simulink model "Processor"  (R2025b)
settings: Solver=VariableStepAuto  StartTime=0.0  StopTime=inf  RelTol=1e-3
libraries: dspsigops x7, hdlsllib x1
settings Model: Creator=cyber  LastModifiedBy=cyber

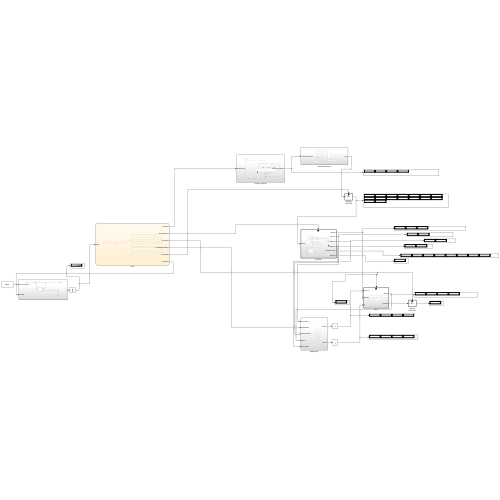
[thumbnail: Simulink's stored preview of the top-level diagram]
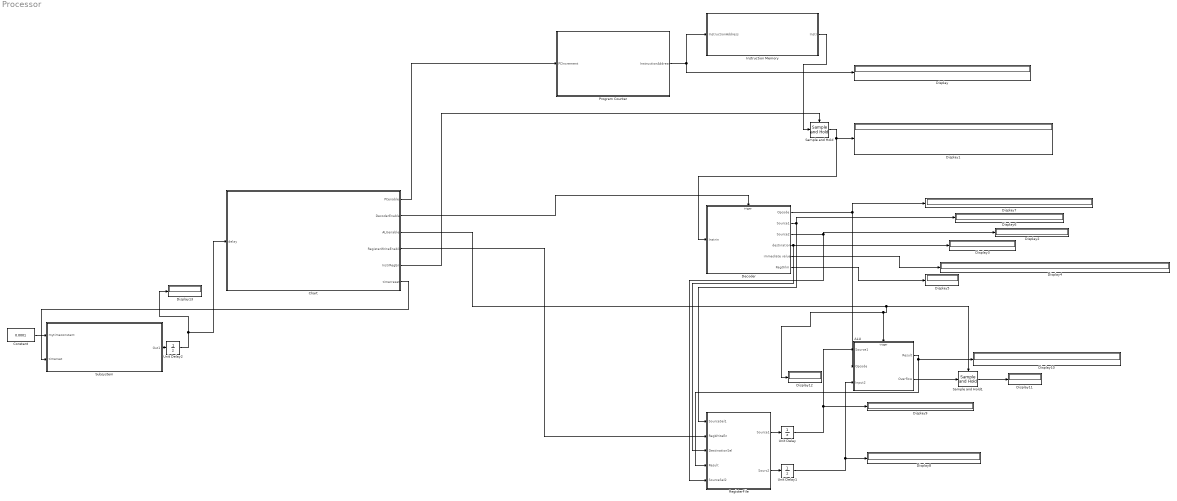
== system Processor ==
  ALU : Subsystem
  Chart : Stateflow chart  TreatAsAtomicUnit=on
  Constant : Constant  Value=0.0001
  Decoder : Subsystem
  Display{,1..13} (14 alike) : Display
  Instruction Memory : Subsystem
  Program Counter : Subsystem
  RegisterFile : Subsystem
  Sample and Hold : dspsigops/Sample and Hold  trig=Rising edge  initCond=0  latchinput=off
  Sample and Hold1 : dspsigops/Sample and Hold  trig=Rising edge  initCond=0  latchinput=off
  Subsystem : Subsystem
  Unit Delay : UnitDelay  SampleTime=-1  HasFrameUpgradeWarning=on
  Unit Delay1 : UnitDelay  SampleTime=-1  HasFrameUpgradeWarning=on
  Unit Delay2 : UnitDelay  SampleTime=-1  HasFrameUpgradeWarning=on
  wires:
  Program Counter/1(InstructionAddress) -> Display/1, Instruction Memory/1(InstructionAddress)
  Instruction Memory/1(Instr) -> Sample and Hold/1
  Sample and Hold/1 -> Decoder/1(Instrin), Display1/1
  Decoder/5(immediate value) -> Display4/1
  Decoder/6(RegOrlm) -> Display5/1
  Decoder/4(destination) -> Display3/1, RegisterFile/3(DestinationSel)
  Decoder/3(Source2) -> RegisterFile/5(SourceSel2), Display2/1
  Decoder/2(Source1) -> RegisterFile/1(SourceSel1), Display6/1
  Decoder/1(Opcode) -> ALU/2(Opcode), Display7/1
  RegisterFile/1(Source1) -> Unit Delay/1
  Unit Delay/1 -> ALU/1(Source1), Display9/1
  RegisterFile/2(Sourc2) -> Unit Delay1/1
  Unit Delay1/1 -> ALU/3(Input2), Display8/1
  ALU/1(Result) -> Display10/1, RegisterFile/4(Result)
  Chart/3(ALUenable) -> Display12/1, ALU/Trigger, Sample and Hold1/Trigger
  ALU/2(Overflow) -> Sample and Hold1/1
  Sample and Hold1/1 -> Display11/1
  Chart/1(PCenable) -> Program Counter/1(PCIncrement)
  Chart/2(DecoderEnable) -> Decoder/Trigger
  Chart/5(InstrRegEn) -> Sample and Hold/Trigger
  Chart/4(RegisterWriteEnable) -> RegisterFile/2(RegWriteEn)
  Subsystem/1(Out1) -> Unit Delay2/1
  Unit Delay2/1 -> Chart/1(delay), Display13/1
  Constant/1 -> Subsystem/1(mytimeconstant)
  Chart/6(timerreset) -> Subsystem/2(timerset)

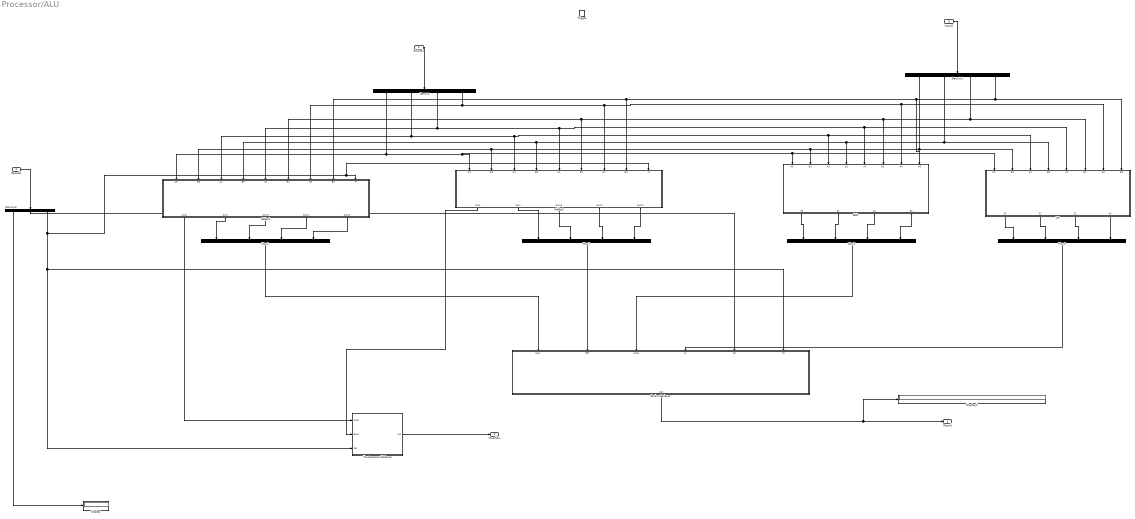
== system Processor/ALU ==
  Source1 : Inport
  Opcode : Inport  Port=2
  Input2 : Inport  Port=3
  Trigger : TriggerPort  VariantControl=(inherit)  PortDimensions=1
  4to1multplexer : Subsystem
  AND : Subsystem
  Adder1 : Subsystem
  Adder2 : Subsystem
  Demux : Demux
  Demux1 : Demux
  Demux2 : Demux  Outputs=3
  Display : Display
  Display1 : Display
  Mux{1..4} (4 alike) : Mux
  OR : Subsystem
  Twotoonemultiplexer : Subsystem
  Result : Outport
  Overflow : Outport  Port=2
  wires:
  Demux2/1 -> Display/1
  Demux1/2 -> OR/4(B2), Adder2/4(B2), Adder1/4(B2), AND/4(B2)
  Mux2/1 -> 4to1multplexer/2(Diff)
  Demux/1 -> Adder1/1(A3), Adder2/1(A3), OR/1(A3), AND/1(A3)
  Adder1/2(Sum) -> Mux1/1
  Demux1/4 -> OR/8(B0), AND/8(B0), Adder2/8(B0), Adder1/8(B0)
  Demux/4 -> Adder1/7(A0), OR/7(A0), AND/7(A0), Adder2/7(A0)
  Demux/2 -> Adder1/3(A2), OR/3(A2), AND/3(A2), Adder2/3(A2)
  Demux1/3 -> OR/6(B1), Adder2/6(B1), Adder1/6(B1), AND/6(B1)
  Demux2/3 -> Adder2/9(M), Adder1/9(M), Twotoonemultiplexer/3(Sel), 4to1multplexer/6(S1)
  Demux1/1 -> OR/2(B3), Adder1/2(B3), Adder2/2(B3), AND/2(B3)
  Demux/3 -> Adder1/5(A1), OR/5(A1), AND/5(A1), Adder2/5(A1)
  Mux4/1 -> 4to1multplexer/4(or)
  Adder2/1(Cout) -> Twotoonemultiplexer/2(Bout)
  Demux2/2 -> 4to1multplexer/5(S0)
  Adder1/3(Sum3) -> Mux1/2
  Mux3/1 -> 4to1multplexer/3(AND)
  Adder1/4(Sum1) -> Mux1/3
  Adder1/1(Cout) -> Twotoonemultiplexer/1(Cout)
  Mux1/1 -> 4to1multplexer/1(Sum)
  Opcode/1 -> Demux2/1
  Twotoonemultiplexer/1(out) -> Overflow/1
  Adder1/5(Sum2) -> Mux1/4
  4to1multplexer/1(out) -> Display1/1, Result/1
  Source1/1 -> Demux/1
  Input2/1 -> Demux1/1
  AND/1(S3) -> Mux3/1
  AND/2(S2) -> Mux3/2
  AND/3(S1) -> Mux3/3
  AND/4(S0) -> Mux3/4
  OR/1(S3) -> Mux4/1
  OR/2(S2) -> Mux4/2
  OR/3(S1) -> Mux4/3
  OR/4(S0) -> Mux4/4
  Adder2/2(Sum) -> Mux2/1
  Adder2/3(Sum3) -> Mux2/2
  Adder2/4(Sum1) -> Mux2/3
  Adder2/5(Sum2) -> Mux2/4

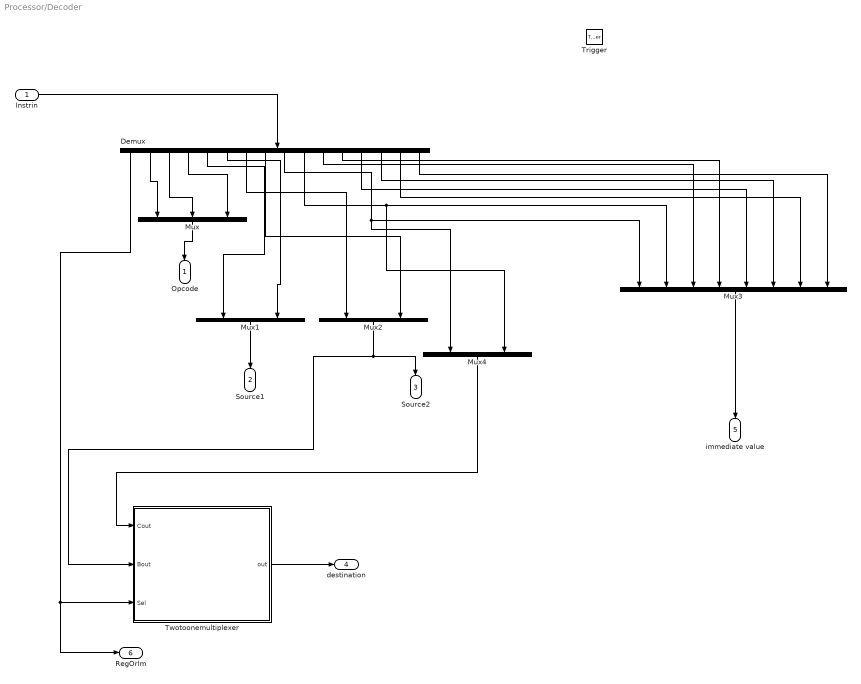
== system Processor/Decoder ==
  Instrin : Inport
  Trigger : TriggerPort  VariantControl=(inherit)  PortDimensions=1
  Demux : Demux  Outputs=16
  Mux : Mux  Inputs=3
  Mux1 : Mux  Inputs=2
  Mux2 : Mux  Inputs=2
  Mux3 : Mux  Inputs=8
  Mux4 : Mux  Inputs=2
  Twotoonemultiplexer : Subsystem
  Opcode : Outport
  Source1 : Outport  Port=2
  Source2 : Outport  Port=3
  destination : Outport  Port=4
  immediate value : Outport  Port=5
  RegOrlm : Outport  Port=6
  wires:
  Demux/12 -> Mux3/4
  Twotoonemultiplexer/1(out) -> destination/1
  Demux/14 -> Mux3/6
  Demux/1 -> RegOrlm/1, Twotoonemultiplexer/3(Sel)
  Mux2/1 -> Source2/1, Twotoonemultiplexer/2(Bout)
  Demux/10 -> Mux4/2, Mux3/2
  Demux/16 -> Mux3/8
  Demux/9 -> Mux4/1, Mux3/1
  Demux/4 -> Mux/3
  Mux4/1 -> Twotoonemultiplexer/1(Cout)
  Demux/8 -> Mux2/2
  Demux/2 -> Mux/1
  Mux3/1 -> immediate value/1
  Demux/7 -> Mux2/1
  Demux/3 -> Mux/2
  Demux/6 -> Mux1/2
  Mux/1 -> Opcode/1
  Mux1/1 -> Source1/1
  Demux/15 -> Mux3/7
  Demux/11 -> Mux3/3
  Demux/13 -> Mux3/5
  Demux/5 -> Mux1/1
  Instrin/1 -> Demux/1

== system Processor/Instruction Memory ==
  InstructionAddress : Inport
  4to1multplexer : Subsystem
  Constant : Constant  Value=[0 0 0 1 0 0 0 1 1 0 0 0 0 0 0 0 ]
  Constant1 : Constant  Value=[0 0 0 0 0 0 0 1 1 0 0 0 0 0 0 0 ]
  Constant2 : Constant  Value=[0 0 0 0 0 0 0 1 1 0 0 0 0 0 0 0 ]
  Constant3 : Constant  Value=[0 0 0 0 0 0 0 1 1 0 0 0 0 0 0 0 ]
  Demux : Demux
  Display : Display
  Display1 : Display
  Display2 : Display
  Instr : Outport
  wires:
  Demux/3 -> 4to1multplexer/5(S0)
  Demux/2 -> Display1/1
  Constant1/1 -> 4to1multplexer/2(2)
  Constant3/1 -> 4to1multplexer/4(4)
  Constant/1 -> 4to1multplexer/1(1)
  4to1multplexer/1(out) -> Instr/1
  Demux/4 -> 4to1multplexer/6(S1)
  Constant2/1 -> 4to1multplexer/3(3)
  InstructionAddress/1 -> Demux/1, Display2/1
  Demux/1 -> Display/1

== system Processor/Program Counter ==
  PCIncrement : Inport
  Adder : Subsystem
  Constant1 : Constant
  Constant2 : Constant  Value=0
  Demux : Demux
  Display : Display
  Mux : Mux
  Program Counter : dspsigops/Sample and Hold  trig=Rising edge  initCond=0  latchinput=off
  Unit Delay : UnitDelay  SampleTime=-1  HasFrameUpgradeWarning=on
  InstructionAddress : Outport
  wires:
  Constant2/1 -> Adder/2(B3), Adder/4(B2), Adder/6(B1), Adder/9(Cin)
  Demux/2 -> Adder/3(A2)
  PCIncrement/1 -> Program Counter/Trigger
  Constant1/1 -> Adder/8(B0)
  Demux/3 -> Adder/5(A1)
  Program Counter/1 -> Demux/1
  Demux/4 -> Adder/7(A0)
  Demux/1 -> Adder/1(A3)
  Adder/2(Sum) -> Mux/1
  Adder/1(Cout) -> Display/1
  Unit Delay/1 -> Program Counter/1
  Mux/1 -> InstructionAddress/1, Unit Delay/1
  Adder/5(Sum2) -> Mux/4
  Adder/3(Sum3) -> Mux/2
  Adder/4(Sum1) -> Mux/3

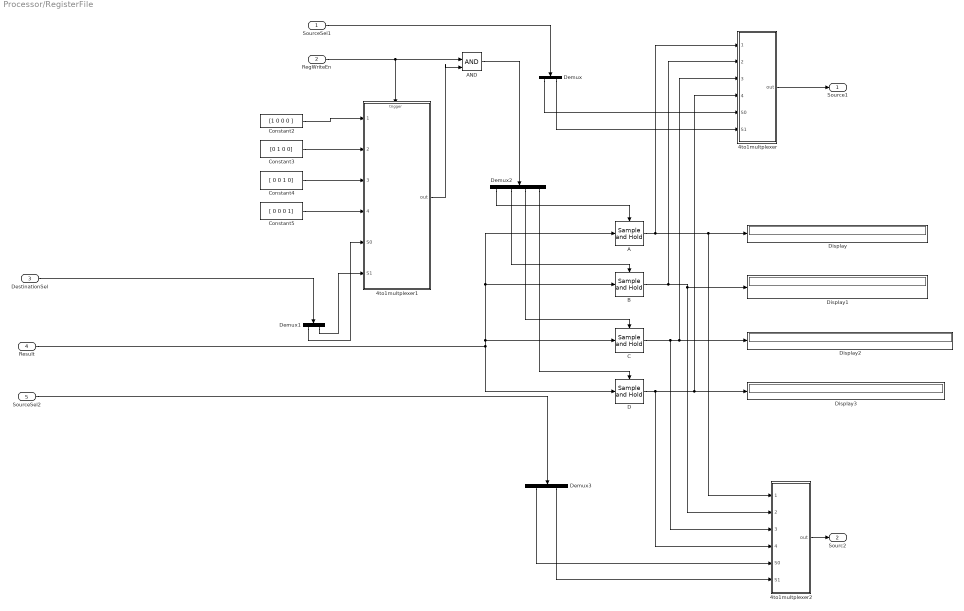
== system Processor/RegisterFile ==
  SourceSel1 : Inport
  RegWriteEn : Inport  Port=2
  DestinationSel : Inport  Port=3
  Result : Inport  Port=4
  SourceSel2 : Inport  Port=5
  4to1multplexer : Subsystem
  4to1multplexer1 : Subsystem
  4to1multplexer2 : Subsystem
  A : dspsigops/Sample and Hold  trig=Rising edge  initCond=[1 0 0 0]  latchinput=off
  AND : Logic  IconShape=distinctive  AllPortsSameDT=off  OutDataTypeStr=boolean
  B : dspsigops/Sample and Hold  trig=Rising edge  initCond=[0 1 0 0]  latchinput=off
  C : dspsigops/Sample and Hold  trig=Rising edge  initCond=[0 0 1 0]  latchinput=off
  Constant2 : Constant  Value=[1 0 0 0 ]
  Constant3 : Constant  Value=[0 1 0 0]
  Constant4 : Constant  Value=[ 0 0 1 0]
  Constant5 : Constant  Value=[ 0 0 0 1]
  D : dspsigops/Sample and Hold  trig=Rising edge  initCond=[0 0 0 1]  latchinput=off
  Demux : Demux  Outputs=2
  Demux1 : Demux  Outputs=2
  Demux2 : Demux
  Demux3 : Demux  Outputs=2
  Display{,1..3} (4 alike) : Display
  Source1 : Outport
  Sourc2 : Outport  Port=2
  wires:
  RegWriteEn/1 -> AND/1, 4to1multplexer1/Trigger
  Demux2/4 -> D/Trigger
  4to1multplexer2/1(out) -> Sourc2/1
  D/1 -> 4to1multplexer2/4(4), Display3/1, 4to1multplexer/4(4)
  C/1 -> 4to1multplexer2/3(3), 4to1multplexer/3(3), Display2/1
  4to1multplexer1/1(out) -> AND/2
  Result/1 -> D/1, A/1, B/1, C/1
  DestinationSel/1 -> Demux1/1
  Constant4/1 -> 4to1multplexer1/3(3)
  Demux3/2 -> 4to1multplexer2/6(S1)
  A/1 -> 4to1multplexer/1(1), 4to1multplexer2/1(1), Display/1
  4to1multplexer/1(out) -> Source1/1
  Demux2/2 -> B/Trigger
  Constant3/1 -> 4to1multplexer1/2(2)
  Demux2/3 -> C/Trigger
  Demux2/1 -> A/Trigger
  AND/1 -> Demux2/1
  Constant5/1 -> 4to1multplexer1/4(4)
  Demux3/1 -> 4to1multplexer2/5(S0)
  Demux/2 -> 4to1multplexer/6(S1)
  SourceSel1/1 -> Demux/1
  Demux1/2 -> 4to1multplexer1/6(S1)
  B/1 -> 4to1multplexer/2(2), 4to1multplexer2/2(2), Display1/1
  SourceSel2/1 -> Demux3/1
  Demux1/1 -> 4to1multplexer1/5(S0)
  Constant2/1 -> 4to1multplexer1/1(1)
  Demux/1 -> 4to1multplexer/5(S0)

== system Processor/Subsystem ==
  mytimeconstant : Inport
  timerset : Inport  Port=2
  Sum : Sum  Inputs=|++
  Unit Delay Resettable Synchronous : hdlsllib/Discrete/Unit Delay Resettable Synchronous  InitialCondition=0.0  SampleTime=-1
  Out1 : Outport
  wires:
  timerset/1 -> Unit Delay Resettable Synchronous/2
  Unit Delay Resettable Synchronous/1 -> Sum/2
  Sum/1 -> Out1/1, Unit Delay Resettable Synchronous/1
  mytimeconstant/1 -> Sum/1

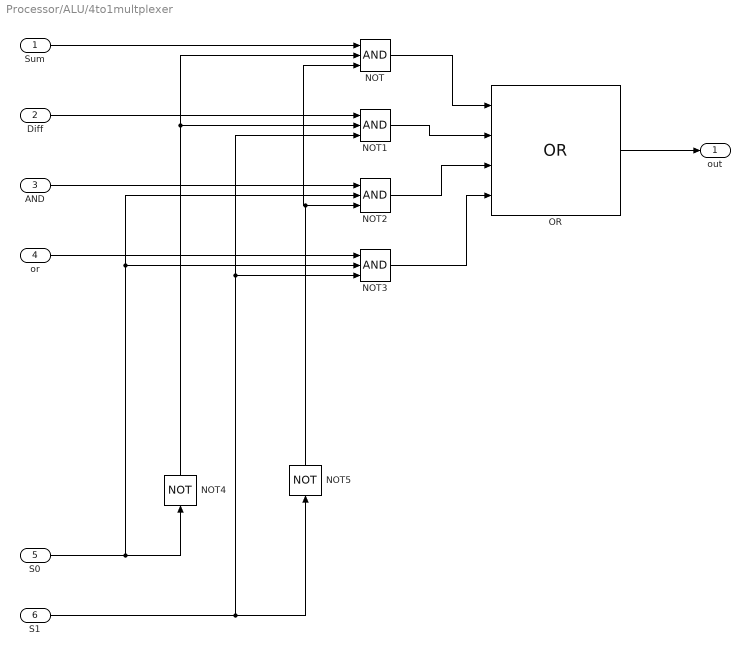
== system Processor/ALU/4to1multplexer ==
  Sum : Inport
  Diff : Inport  Port=2
  AND : Inport  Port=3
  or : Inport  Port=4
  S0 : Inport  Port=5
  S1 : Inport  Port=6
  NOT{,1..3} (4 alike) : Logic  Inputs=3  IconShape=distinctive  AllPortsSameDT=off  OutDataTypeStr=boolean
  NOT4 : Logic  Operator=NOT  IconShape=distinctive  AllPortsSameDT=off  OutDataTypeStr=boolean
  NOT5 : Logic  Operator=NOT  IconShape=distinctive  AllPortsSameDT=off  OutDataTypeStr=boolean
  OR : Logic  Operator=OR  Inputs=4  IconShape=distinctive  AllPortsSameDT=off  OutDataTypeStr=boolean
  out : Outport
  wires:
  NOT4/1 -> NOT/2, NOT1/2
  S1/1 -> NOT1/3, NOT3/3, NOT5/1
  NOT5/1 -> NOT/3, NOT2/3
  NOT1/1 -> OR/2
  S0/1 -> NOT4/1, NOT3/2, NOT2/2
  NOT3/1 -> OR/4
  NOT/1 -> OR/1
  NOT2/1 -> OR/3
  or/1 -> NOT3/1
  Sum/1 -> NOT/1
  AND/1 -> NOT2/1
  Diff/1 -> NOT1/1
  OR/1 -> out/1

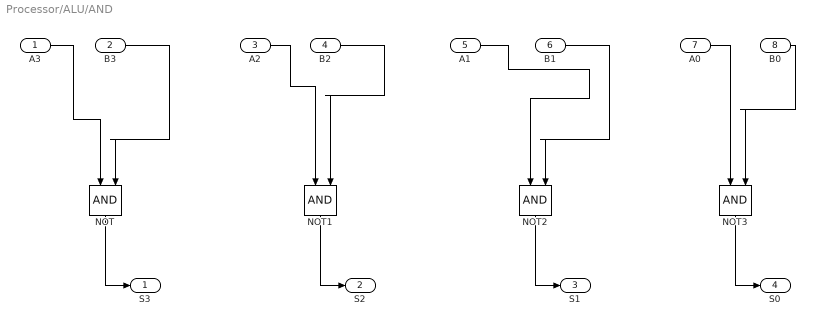
== system Processor/ALU/AND ==
  A3 : Inport
  B3 : Inport  Port=2
  A2 : Inport  Port=3
  B2 : Inport  Port=4
  A1 : Inport  Port=5
  B1 : Inport  Port=6
  A0 : Inport  Port=7
  B0 : Inport  Port=8
  NOT{,1..3} (4 alike) : Logic  IconShape=distinctive  AllPortsSameDT=off  OutDataTypeStr=boolean
  S3 : Outport
  S2 : Outport  Port=2
  S1 : Outport  Port=3
  S0 : Outport  Port=4
  wires:
  B0/1 -> NOT3/2
  NOT/1 -> S3/1
  NOT1/1 -> S2/1
  B1/1 -> NOT2/2
  NOT3/1 -> S0/1
  A3/1 -> NOT/1
  NOT2/1 -> S1/1
  A0/1 -> NOT3/1
  B2/1 -> NOT1/2
  A2/1 -> NOT1/1
  B3/1 -> NOT/2
  A1/1 -> NOT2/1

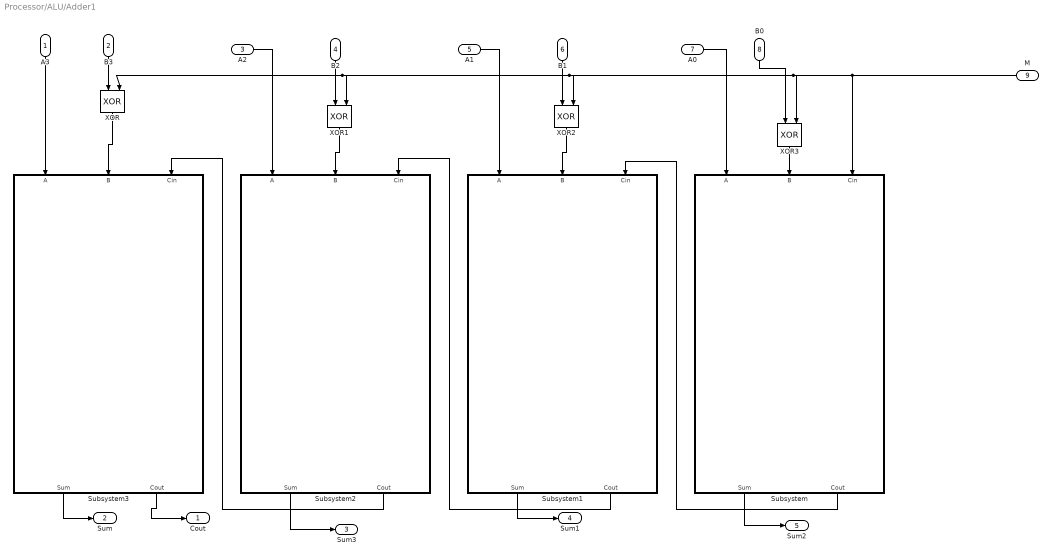
== system Processor/ALU/Adder1 ==
  A3 : Inport
  B3 : Inport  Port=2
  A2 : Inport  Port=3
  B2 : Inport  Port=4
  A1 : Inport  Port=5
  B1 : Inport  Port=6
  A0 : Inport  Port=7
  B0 : Inport  Port=8
  M : Inport  Port=9
  Subsystem : Subsystem
  Subsystem1 : Subsystem
  Subsystem2 : Subsystem
  Subsystem3 : Subsystem
  XOR{,1..3} (4 alike) : Logic  Operator=XOR  IconShape=distinctive  AllPortsSameDT=off  OutDataTypeStr=boolean
  Cout : Outport
  Sum : Outport  Port=2
  Sum3 : Outport  Port=3
  Sum1 : Outport  Port=4
  Sum2 : Outport  Port=5
  wires:
  Subsystem2/2(Cout) -> Subsystem3/3(Cin)
  Subsystem/2(Cout) -> Subsystem1/3(Cin)
  A2/1 -> Subsystem2/1(A)
  A3/1 -> Subsystem3/1(A)
  A1/1 -> Subsystem1/1(A)
  Subsystem/1(Sum) -> Sum2/1
  Subsystem1/2(Cout) -> Subsystem2/3(Cin)
  Subsystem3/1(Sum) -> Sum/1
  Subsystem1/1(Sum) -> Sum1/1
  Subsystem2/1(Sum) -> Sum3/1
  M/1 -> Subsystem/3(Cin), XOR3/2, XOR2/2, XOR1/2, XOR/2
  Subsystem3/2(Cout) -> Cout/1
  A0/1 -> Subsystem/1(A)
  B3/1 -> XOR/1
  XOR/1 -> Subsystem3/2(B)
  B2/1 -> XOR1/1
  XOR1/1 -> Subsystem2/2(B)
  B1/1 -> XOR2/1
  XOR2/1 -> Subsystem1/2(B)
  XOR3/1 -> Subsystem/2(B)
  B0/1 -> XOR3/1

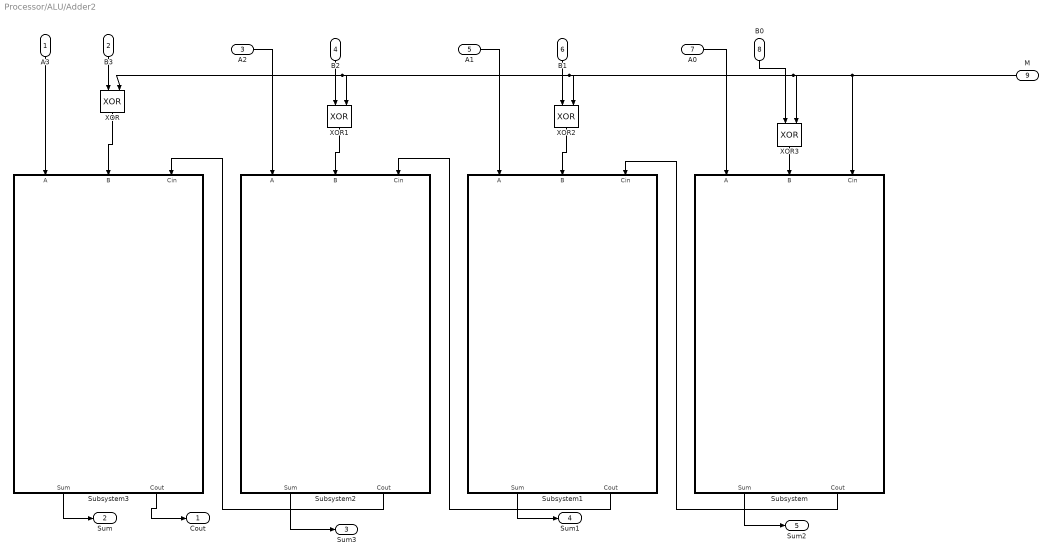
== system Processor/ALU/Adder2 ==
  A3 : Inport
  B3 : Inport  Port=2
  A2 : Inport  Port=3
  B2 : Inport  Port=4
  A1 : Inport  Port=5
  B1 : Inport  Port=6
  A0 : Inport  Port=7
  B0 : Inport  Port=8
  M : Inport  Port=9
  Subsystem : Subsystem
  Subsystem1 : Subsystem
  Subsystem2 : Subsystem
  Subsystem3 : Subsystem
  XOR{,1..3} (4 alike) : Logic  Operator=XOR  IconShape=distinctive  AllPortsSameDT=off  OutDataTypeStr=boolean
  Cout : Outport
  Sum : Outport  Port=2
  Sum3 : Outport  Port=3
  Sum1 : Outport  Port=4
  Sum2 : Outport  Port=5
  wires:
  Subsystem2/2(Cout) -> Subsystem3/3(Cin)
  Subsystem/2(Cout) -> Subsystem1/3(Cin)
  A2/1 -> Subsystem2/1(A)
  A3/1 -> Subsystem3/1(A)
  A1/1 -> Subsystem1/1(A)
  Subsystem/1(Sum) -> Sum2/1
  Subsystem1/2(Cout) -> Subsystem2/3(Cin)
  Subsystem3/1(Sum) -> Sum/1
  Subsystem1/1(Sum) -> Sum1/1
  Subsystem2/1(Sum) -> Sum3/1
  M/1 -> Subsystem/3(Cin), XOR3/2, XOR2/2, XOR1/2, XOR/2
  Subsystem3/2(Cout) -> Cout/1
  A0/1 -> Subsystem/1(A)
  B3/1 -> XOR/1
  XOR/1 -> Subsystem3/2(B)
  B2/1 -> XOR1/1
  XOR1/1 -> Subsystem2/2(B)
  B1/1 -> XOR2/1
  XOR2/1 -> Subsystem1/2(B)
  XOR3/1 -> Subsystem/2(B)
  B0/1 -> XOR3/1

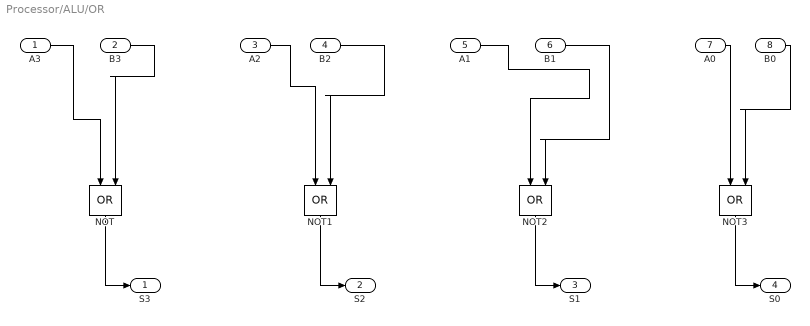
== system Processor/ALU/OR ==
  A3 : Inport
  B3 : Inport  Port=2
  A2 : Inport  Port=3
  B2 : Inport  Port=4
  A1 : Inport  Port=5
  B1 : Inport  Port=6
  A0 : Inport  Port=7
  B0 : Inport  Port=8
  NOT{,1..3} (4 alike) : Logic  Operator=OR  IconShape=distinctive  AllPortsSameDT=off  OutDataTypeStr=boolean
  S3 : Outport
  S2 : Outport  Port=2
  S1 : Outport  Port=3
  S0 : Outport  Port=4
  wires:
  B3/1 -> NOT/2
  B0/1 -> NOT3/2
  A0/1 -> NOT3/1
  NOT3/1 -> S0/1
  A3/1 -> NOT/1
  NOT/1 -> S3/1
  A1/1 -> NOT2/1
  NOT1/1 -> S2/1
  NOT2/1 -> S1/1
  A2/1 -> NOT1/1
  B1/1 -> NOT2/2
  B2/1 -> NOT1/2

== system Processor/ALU/Twotoonemultiplexer ==
  Cout : Inport
  Bout : Inport  Port=2
  Sel : Inport  Port=3
  NOT : Logic  IconShape=distinctive  AllPortsSameDT=off  OutDataTypeStr=boolean
  NOT1 : Logic  IconShape=distinctive  AllPortsSameDT=off  OutDataTypeStr=boolean
  NOT2 : Logic  Operator=NOT  IconShape=distinctive  AllPortsSameDT=off  OutDataTypeStr=boolean
  NOT3 : Logic  Operator=OR  IconShape=distinctive  AllPortsSameDT=off  OutDataTypeStr=boolean
  out : Outport
  wires:
  Cout/1 -> NOT/1
  Sel/1 -> NOT1/2, NOT2/1
  NOT1/1 -> NOT3/2
  Bout/1 -> NOT1/1
  NOT2/1 -> NOT/2
  NOT/1 -> NOT3/1
  NOT3/1 -> out/1

== system Processor/Decoder/Twotoonemultiplexer ==
  Cout : Inport
  Bout : Inport  Port=2
  Sel : Inport  Port=3
  NOT : Logic  IconShape=distinctive  AllPortsSameDT=off  OutDataTypeStr=boolean
  NOT1 : Logic  IconShape=distinctive  AllPortsSameDT=off  OutDataTypeStr=boolean
  NOT2 : Logic  Operator=NOT  IconShape=distinctive  AllPortsSameDT=off  OutDataTypeStr=boolean
  NOT3 : Logic  Operator=OR  IconShape=distinctive  AllPortsSameDT=off  OutDataTypeStr=boolean
  out : Outport
  wires:
  Cout/1 -> NOT/1
  Sel/1 -> NOT1/2, NOT2/1
  NOT1/1 -> NOT3/2
  Bout/1 -> NOT1/1
  NOT2/1 -> NOT/2
  NOT/1 -> NOT3/1
  NOT3/1 -> out/1

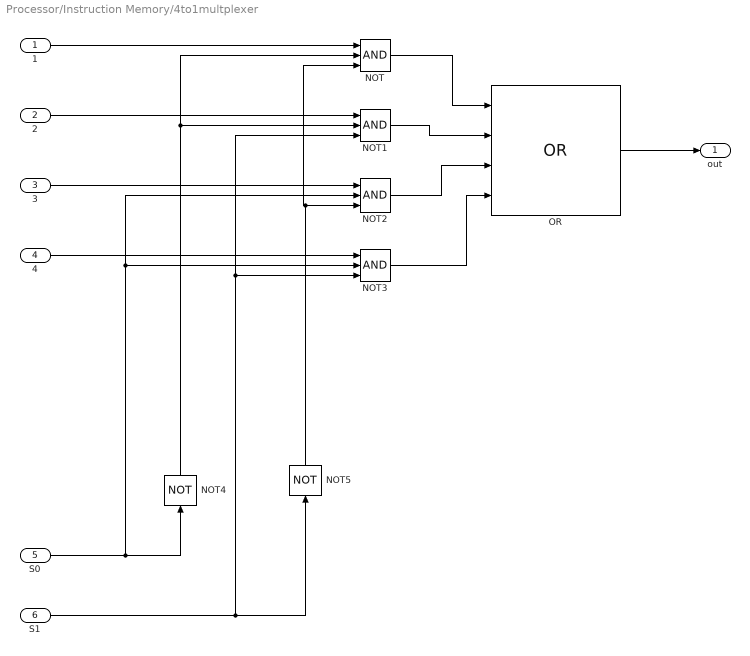
== system Processor/Instruction Memory/4to1multplexer ==
  1 : Inport
  2 : Inport  Port=2
  3 : Inport  Port=3
  4 : Inport  Port=4
  S0 : Inport  Port=5
  S1 : Inport  Port=6
  NOT{,1..3} (4 alike) : Logic  Inputs=3  IconShape=distinctive  AllPortsSameDT=off  OutDataTypeStr=boolean
  NOT4 : Logic  Operator=NOT  IconShape=distinctive  AllPortsSameDT=off  OutDataTypeStr=boolean
  NOT5 : Logic  Operator=NOT  IconShape=distinctive  AllPortsSameDT=off  OutDataTypeStr=boolean
  OR : Logic  Operator=OR  Inputs=4  IconShape=distinctive  AllPortsSameDT=off  OutDataTypeStr=boolean
  out : Outport
  wires:
  NOT4/1 -> NOT/2, NOT1/2
  S1/1 -> NOT1/3, NOT3/3, NOT5/1
  NOT5/1 -> NOT/3, NOT2/3
  NOT1/1 -> OR/2
  S0/1 -> NOT4/1, NOT3/2, NOT2/2
  NOT3/1 -> OR/4
  NOT/1 -> OR/1
  NOT2/1 -> OR/3
  4/1 -> NOT3/1
  1/1 -> NOT/1
  3/1 -> NOT2/1
  2/1 -> NOT1/1
  OR/1 -> out/1

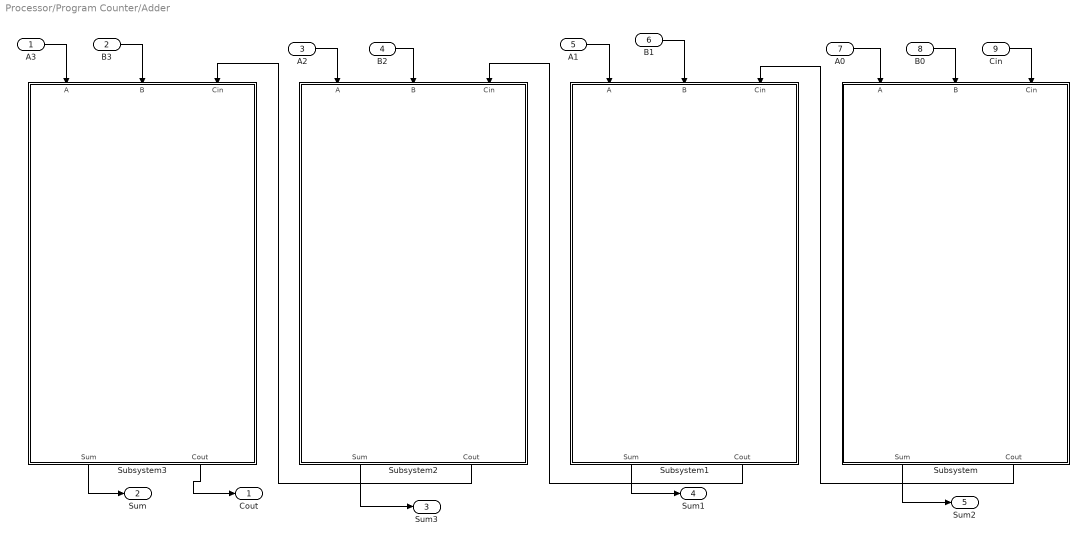
== system Processor/Program Counter/Adder ==
  A3 : Inport
  B3 : Inport  Port=2
  A2 : Inport  Port=3
  B2 : Inport  Port=4
  A1 : Inport  Port=5
  B1 : Inport  Port=6
  A0 : Inport  Port=7
  B0 : Inport  Port=8
  Cin : Inport  Port=9
  Subsystem : Subsystem
  Subsystem1 : Subsystem
  Subsystem2 : Subsystem
  Subsystem3 : Subsystem
  Cout : Outport
  Sum : Outport  Port=2
  Sum3 : Outport  Port=3
  Sum1 : Outport  Port=4
  Sum2 : Outport  Port=5
  wires:
  Subsystem2/2(Cout) -> Subsystem3/3(Cin)
  B3/1 -> Subsystem3/2(B)
  Subsystem/2(Cout) -> Subsystem1/3(Cin)
  A2/1 -> Subsystem2/1(A)
  A3/1 -> Subsystem3/1(A)
  A1/1 -> Subsystem1/1(A)
  Subsystem/1(Sum) -> Sum2/1
  Subsystem1/2(Cout) -> Subsystem2/3(Cin)
  B1/1 -> Subsystem1/2(B)
  B0/1 -> Subsystem/2(B)
  Subsystem3/1(Sum) -> Sum/1
  B2/1 -> Subsystem2/2(B)
  Subsystem1/1(Sum) -> Sum1/1
  Subsystem2/1(Sum) -> Sum3/1
  Cin/1 -> Subsystem/3(Cin)
  Subsystem3/2(Cout) -> Cout/1
  A0/1 -> Subsystem/1(A)

== system Processor/RegisterFile/4to1multplexer ==
  1 : Inport
  2 : Inport  Port=2
  3 : Inport  Port=3
  4 : Inport  Port=4
  S0 : Inport  Port=5
  S1 : Inport  Port=6
  NOT{,1..3} (4 alike) : Logic  Inputs=3  IconShape=distinctive  AllPortsSameDT=off  OutDataTypeStr=boolean
  NOT4 : Logic  Operator=NOT  IconShape=distinctive  AllPortsSameDT=off  OutDataTypeStr=boolean
  NOT5 : Logic  Operator=NOT  IconShape=distinctive  AllPortsSameDT=off  OutDataTypeStr=boolean
  OR : Logic  Operator=OR  Inputs=4  IconShape=distinctive  AllPortsSameDT=off  OutDataTypeStr=boolean
  out : Outport
  wires:
  NOT4/1 -> NOT/2, NOT1/2
  S1/1 -> NOT1/3, NOT3/3, NOT5/1
  NOT5/1 -> NOT/3, NOT2/3
  NOT1/1 -> OR/2
  S0/1 -> NOT4/1, NOT3/2, NOT2/2
  NOT3/1 -> OR/4
  NOT/1 -> OR/1
  NOT2/1 -> OR/3
  4/1 -> NOT3/1
  1/1 -> NOT/1
  3/1 -> NOT2/1
  2/1 -> NOT1/1
  OR/1 -> out/1

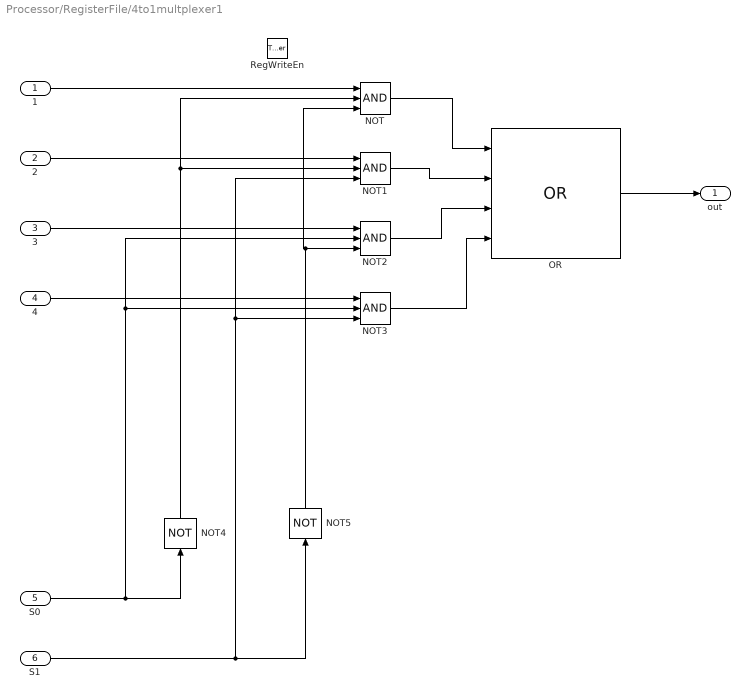
== system Processor/RegisterFile/4to1multplexer1 ==
  1 : Inport
  2 : Inport  Port=2
  3 : Inport  Port=3
  4 : Inport  Port=4
  S0 : Inport  Port=5
  S1 : Inport  Port=6
  RegWriteEn : TriggerPort  VariantControl=(inherit)  PortDimensions=1
  NOT{,1..3} (4 alike) : Logic  Inputs=3  IconShape=distinctive  AllPortsSameDT=off  OutDataTypeStr=boolean
  NOT4 : Logic  Operator=NOT  IconShape=distinctive  AllPortsSameDT=off  OutDataTypeStr=boolean
  NOT5 : Logic  Operator=NOT  IconShape=distinctive  AllPortsSameDT=off  OutDataTypeStr=boolean
  OR : Logic  Operator=OR  Inputs=4  IconShape=distinctive  AllPortsSameDT=off  OutDataTypeStr=boolean
  out : Outport
  wires:
  NOT4/1 -> NOT/2, NOT1/2
  S1/1 -> NOT1/3, NOT3/3, NOT5/1
  NOT5/1 -> NOT/3, NOT2/3
  NOT1/1 -> OR/2
  S0/1 -> NOT4/1, NOT3/2, NOT2/2
  NOT3/1 -> OR/4
  NOT/1 -> OR/1
  NOT2/1 -> OR/3
  4/1 -> NOT3/1
  1/1 -> NOT/1
  3/1 -> NOT2/1
  2/1 -> NOT1/1
  OR/1 -> out/1

== system Processor/RegisterFile/4to1multplexer2 ==
  1 : Inport
  2 : Inport  Port=2
  3 : Inport  Port=3
  4 : Inport  Port=4
  S0 : Inport  Port=5
  S1 : Inport  Port=6
  NOT{,1..3} (4 alike) : Logic  Inputs=3  IconShape=distinctive  AllPortsSameDT=off  OutDataTypeStr=boolean
  NOT4 : Logic  Operator=NOT  IconShape=distinctive  AllPortsSameDT=off  OutDataTypeStr=boolean
  NOT5 : Logic  Operator=NOT  IconShape=distinctive  AllPortsSameDT=off  OutDataTypeStr=boolean
  OR : Logic  Operator=OR  Inputs=4  IconShape=distinctive  AllPortsSameDT=off  OutDataTypeStr=boolean
  out : Outport
  wires:
  NOT4/1 -> NOT/2, NOT1/2
  S1/1 -> NOT1/3, NOT3/3, NOT5/1
  NOT5/1 -> NOT/3, NOT2/3
  NOT1/1 -> OR/2
  S0/1 -> NOT4/1, NOT3/2, NOT2/2
  NOT3/1 -> OR/4
  NOT/1 -> OR/1
  NOT2/1 -> OR/3
  4/1 -> NOT3/1
  1/1 -> NOT/1
  3/1 -> NOT2/1
  2/1 -> NOT1/1
  OR/1 -> out/1

== system Processor/ALU/Adder1/Subsystem ==
  A : Inport
  B : Inport  Port=2
  Cin : Inport  Port=3
  Logical Operator : Logic  Operator=XOR  IconShape=distinctive  AllPortsSameDT=off  OutDataTypeStr=boolean
  Logical Operator1 : Logic  Operator=XOR  IconShape=distinctive  AllPortsSameDT=off  OutDataTypeStr=boolean
  Logical Operator2 : Logic  IconShape=distinctive  AllPortsSameDT=off  OutDataTypeStr=boolean
  Logical Operator3 : Logic  IconShape=distinctive  AllPortsSameDT=off  OutDataTypeStr=boolean
  Logical Operator4 : Logic  Operator=OR  IconShape=distinctive  AllPortsSameDT=off  OutDataTypeStr=boolean
  Sum : Outport
  Cout : Outport  Port=2
  wires:
  B/1 -> Logical Operator3/1, Logical Operator/2
  Logical Operator1/1 -> Sum/1
  Logical Operator3/1 -> Logical Operator4/2
  Logical Operator/1 -> Logical Operator2/2, Logical Operator1/1
  Logical Operator4/1 -> Cout/1
  Cin/1 -> Logical Operator2/1, Logical Operator1/2
  Logical Operator2/1 -> Logical Operator4/1
  A/1 -> Logical Operator3/2, Logical Operator/1

== system Processor/ALU/Adder1/Subsystem1 ==
  A : Inport
  B : Inport  Port=2
  Cin : Inport  Port=3
  Logical Operator : Logic  Operator=XOR  IconShape=distinctive  AllPortsSameDT=off  OutDataTypeStr=boolean
  Logical Operator1 : Logic  Operator=XOR  IconShape=distinctive  AllPortsSameDT=off  OutDataTypeStr=boolean
  Logical Operator2 : Logic  IconShape=distinctive  AllPortsSameDT=off  OutDataTypeStr=boolean
  Logical Operator3 : Logic  IconShape=distinctive  AllPortsSameDT=off  OutDataTypeStr=boolean
  Logical Operator4 : Logic  Operator=OR  IconShape=distinctive  AllPortsSameDT=off  OutDataTypeStr=boolean
  Sum : Outport
  Cout : Outport  Port=2
  wires:
  B/1 -> Logical Operator3/1, Logical Operator/2
  Logical Operator1/1 -> Sum/1
  Logical Operator3/1 -> Logical Operator4/2
  Logical Operator/1 -> Logical Operator2/2, Logical Operator1/1
  Logical Operator4/1 -> Cout/1
  Cin/1 -> Logical Operator2/1, Logical Operator1/2
  Logical Operator2/1 -> Logical Operator4/1
  A/1 -> Logical Operator3/2, Logical Operator/1

== system Processor/ALU/Adder1/Subsystem2 ==
  A : Inport
  B : Inport  Port=2
  Cin : Inport  Port=3
  Logical Operator : Logic  Operator=XOR  IconShape=distinctive  AllPortsSameDT=off  OutDataTypeStr=boolean
  Logical Operator1 : Logic  Operator=XOR  IconShape=distinctive  AllPortsSameDT=off  OutDataTypeStr=boolean
  Logical Operator2 : Logic  IconShape=distinctive  AllPortsSameDT=off  OutDataTypeStr=boolean
  Logical Operator3 : Logic  IconShape=distinctive  AllPortsSameDT=off  OutDataTypeStr=boolean
  Logical Operator4 : Logic  Operator=OR  IconShape=distinctive  AllPortsSameDT=off  OutDataTypeStr=boolean
  Sum : Outport
  Cout : Outport  Port=2
  wires:
  B/1 -> Logical Operator3/1, Logical Operator/2
  Logical Operator1/1 -> Sum/1
  Logical Operator3/1 -> Logical Operator4/2
  Logical Operator/1 -> Logical Operator2/2, Logical Operator1/1
  Logical Operator4/1 -> Cout/1
  Cin/1 -> Logical Operator2/1, Logical Operator1/2
  Logical Operator2/1 -> Logical Operator4/1
  A/1 -> Logical Operator3/2, Logical Operator/1

== system Processor/ALU/Adder1/Subsystem3 ==
  A : Inport
  B : Inport  Port=2
  Cin : Inport  Port=3
  Logical Operator : Logic  Operator=XOR  IconShape=distinctive  AllPortsSameDT=off  OutDataTypeStr=boolean
  Logical Operator1 : Logic  Operator=XOR  IconShape=distinctive  AllPortsSameDT=off  OutDataTypeStr=boolean
  Logical Operator2 : Logic  IconShape=distinctive  AllPortsSameDT=off  OutDataTypeStr=boolean
  Logical Operator3 : Logic  IconShape=distinctive  AllPortsSameDT=off  OutDataTypeStr=boolean
  Logical Operator4 : Logic  Operator=OR  IconShape=distinctive  AllPortsSameDT=off  OutDataTypeStr=boolean
  Sum : Outport
  Cout : Outport  Port=2
  wires:
  B/1 -> Logical Operator3/1, Logical Operator/2
  Logical Operator1/1 -> Sum/1
  Logical Operator3/1 -> Logical Operator4/2
  Logical Operator/1 -> Logical Operator2/2, Logical Operator1/1
  Logical Operator4/1 -> Cout/1
  Cin/1 -> Logical Operator2/1, Logical Operator1/2
  Logical Operator2/1 -> Logical Operator4/1
  A/1 -> Logical Operator3/2, Logical Operator/1

== system Processor/ALU/Adder2/Subsystem ==
  A : Inport
  B : Inport  Port=2
  Cin : Inport  Port=3
  Logical Operator : Logic  Operator=XOR  IconShape=distinctive  AllPortsSameDT=off  OutDataTypeStr=boolean
  Logical Operator1 : Logic  Operator=XOR  IconShape=distinctive  AllPortsSameDT=off  OutDataTypeStr=boolean
  Logical Operator2 : Logic  IconShape=distinctive  AllPortsSameDT=off  OutDataTypeStr=boolean
  Logical Operator3 : Logic  IconShape=distinctive  AllPortsSameDT=off  OutDataTypeStr=boolean
  Logical Operator4 : Logic  Operator=OR  IconShape=distinctive  AllPortsSameDT=off  OutDataTypeStr=boolean
  Sum : Outport
  Cout : Outport  Port=2
  wires:
  B/1 -> Logical Operator3/1, Logical Operator/2
  Logical Operator1/1 -> Sum/1
  Logical Operator3/1 -> Logical Operator4/2
  Logical Operator/1 -> Logical Operator2/2, Logical Operator1/1
  Logical Operator4/1 -> Cout/1
  Cin/1 -> Logical Operator2/1, Logical Operator1/2
  Logical Operator2/1 -> Logical Operator4/1
  A/1 -> Logical Operator3/2, Logical Operator/1

== system Processor/ALU/Adder2/Subsystem1 ==
  A : Inport
  B : Inport  Port=2
  Cin : Inport  Port=3
  Logical Operator : Logic  Operator=XOR  IconShape=distinctive  AllPortsSameDT=off  OutDataTypeStr=boolean
  Logical Operator1 : Logic  Operator=XOR  IconShape=distinctive  AllPortsSameDT=off  OutDataTypeStr=boolean
  Logical Operator2 : Logic  IconShape=distinctive  AllPortsSameDT=off  OutDataTypeStr=boolean
  Logical Operator3 : Logic  IconShape=distinctive  AllPortsSameDT=off  OutDataTypeStr=boolean
  Logical Operator4 : Logic  Operator=OR  IconShape=distinctive  AllPortsSameDT=off  OutDataTypeStr=boolean
  Sum : Outport
  Cout : Outport  Port=2
  wires:
  B/1 -> Logical Operator3/1, Logical Operator/2
  Logical Operator1/1 -> Sum/1
  Logical Operator3/1 -> Logical Operator4/2
  Logical Operator/1 -> Logical Operator2/2, Logical Operator1/1
  Logical Operator4/1 -> Cout/1
  Cin/1 -> Logical Operator2/1, Logical Operator1/2
  Logical Operator2/1 -> Logical Operator4/1
  A/1 -> Logical Operator3/2, Logical Operator/1

== system Processor/ALU/Adder2/Subsystem2 ==
  A : Inport
  B : Inport  Port=2
  Cin : Inport  Port=3
  Logical Operator : Logic  Operator=XOR  IconShape=distinctive  AllPortsSameDT=off  OutDataTypeStr=boolean
  Logical Operator1 : Logic  Operator=XOR  IconShape=distinctive  AllPortsSameDT=off  OutDataTypeStr=boolean
  Logical Operator2 : Logic  IconShape=distinctive  AllPortsSameDT=off  OutDataTypeStr=boolean
  Logical Operator3 : Logic  IconShape=distinctive  AllPortsSameDT=off  OutDataTypeStr=boolean
  Logical Operator4 : Logic  Operator=OR  IconShape=distinctive  AllPortsSameDT=off  OutDataTypeStr=boolean
  Sum : Outport
  Cout : Outport  Port=2
  wires:
  B/1 -> Logical Operator3/1, Logical Operator/2
  Logical Operator1/1 -> Sum/1
  Logical Operator3/1 -> Logical Operator4/2
  Logical Operator/1 -> Logical Operator2/2, Logical Operator1/1
  Logical Operator4/1 -> Cout/1
  Cin/1 -> Logical Operator2/1, Logical Operator1/2
  Logical Operator2/1 -> Logical Operator4/1
  A/1 -> Logical Operator3/2, Logical Operator/1

== system Processor/ALU/Adder2/Subsystem3 ==
  A : Inport
  B : Inport  Port=2
  Cin : Inport  Port=3
  Logical Operator : Logic  Operator=XOR  IconShape=distinctive  AllPortsSameDT=off  OutDataTypeStr=boolean
  Logical Operator1 : Logic  Operator=XOR  IconShape=distinctive  AllPortsSameDT=off  OutDataTypeStr=boolean
  Logical Operator2 : Logic  IconShape=distinctive  AllPortsSameDT=off  OutDataTypeStr=boolean
  Logical Operator3 : Logic  IconShape=distinctive  AllPortsSameDT=off  OutDataTypeStr=boolean
  Logical Operator4 : Logic  Operator=OR  IconShape=distinctive  AllPortsSameDT=off  OutDataTypeStr=boolean
  Sum : Outport
  Cout : Outport  Port=2
  wires:
  B/1 -> Logical Operator3/1, Logical Operator/2
  Logical Operator1/1 -> Sum/1
  Logical Operator3/1 -> Logical Operator4/2
  Logical Operator/1 -> Logical Operator2/2, Logical Operator1/1
  Logical Operator4/1 -> Cout/1
  Cin/1 -> Logical Operator2/1, Logical Operator1/2
  Logical Operator2/1 -> Logical Operator4/1
  A/1 -> Logical Operator3/2, Logical Operator/1

== system Processor/Program Counter/Adder/Subsystem ==
  A : Inport
  B : Inport  Port=2
  Cin : Inport  Port=3
  Logical Operator : Logic  Operator=XOR  IconShape=distinctive  AllPortsSameDT=off  OutDataTypeStr=boolean
  Logical Operator1 : Logic  Operator=XOR  IconShape=distinctive  AllPortsSameDT=off  OutDataTypeStr=boolean
  Logical Operator2 : Logic  IconShape=distinctive  AllPortsSameDT=off  OutDataTypeStr=boolean
  Logical Operator3 : Logic  IconShape=distinctive  AllPortsSameDT=off  OutDataTypeStr=boolean
  Logical Operator4 : Logic  Operator=OR  IconShape=distinctive  AllPortsSameDT=off  OutDataTypeStr=boolean
  Sum : Outport
  Cout : Outport  Port=2
  wires:
  B/1 -> Logical Operator3/1, Logical Operator/2
  Logical Operator1/1 -> Sum/1
  Logical Operator3/1 -> Logical Operator4/2
  Logical Operator/1 -> Logical Operator2/2, Logical Operator1/1
  Logical Operator4/1 -> Cout/1
  Cin/1 -> Logical Operator2/1, Logical Operator1/2
  Logical Operator2/1 -> Logical Operator4/1
  A/1 -> Logical Operator3/2, Logical Operator/1

== system Processor/Program Counter/Adder/Subsystem1 ==
  A : Inport
  B : Inport  Port=2
  Cin : Inport  Port=3
  Logical Operator : Logic  Operator=XOR  IconShape=distinctive  AllPortsSameDT=off  OutDataTypeStr=boolean
  Logical Operator1 : Logic  Operator=XOR  IconShape=distinctive  AllPortsSameDT=off  OutDataTypeStr=boolean
  Logical Operator2 : Logic  IconShape=distinctive  AllPortsSameDT=off  OutDataTypeStr=boolean
  Logical Operator3 : Logic  IconShape=distinctive  AllPortsSameDT=off  OutDataTypeStr=boolean
  Logical Operator4 : Logic  Operator=OR  IconShape=distinctive  AllPortsSameDT=off  OutDataTypeStr=boolean
  Sum : Outport
  Cout : Outport  Port=2
  wires:
  B/1 -> Logical Operator3/1, Logical Operator/2
  Logical Operator1/1 -> Sum/1
  Logical Operator3/1 -> Logical Operator4/2
  Logical Operator/1 -> Logical Operator2/2, Logical Operator1/1
  Logical Operator4/1 -> Cout/1
  Cin/1 -> Logical Operator2/1, Logical Operator1/2
  Logical Operator2/1 -> Logical Operator4/1
  A/1 -> Logical Operator3/2, Logical Operator/1

== system Processor/Program Counter/Adder/Subsystem2 ==
  A : Inport
  B : Inport  Port=2
  Cin : Inport  Port=3
  Logical Operator : Logic  Operator=XOR  IconShape=distinctive  AllPortsSameDT=off  OutDataTypeStr=boolean
  Logical Operator1 : Logic  Operator=XOR  IconShape=distinctive  AllPortsSameDT=off  OutDataTypeStr=boolean
  Logical Operator2 : Logic  IconShape=distinctive  AllPortsSameDT=off  OutDataTypeStr=boolean
  Logical Operator3 : Logic  IconShape=distinctive  AllPortsSameDT=off  OutDataTypeStr=boolean
  Logical Operator4 : Logic  Operator=OR  IconShape=distinctive  AllPortsSameDT=off  OutDataTypeStr=boolean
  Sum : Outport
  Cout : Outport  Port=2
  wires:
  B/1 -> Logical Operator3/1, Logical Operator/2
  Logical Operator1/1 -> Sum/1
  Logical Operator3/1 -> Logical Operator4/2
  Logical Operator/1 -> Logical Operator2/2, Logical Operator1/1
  Logical Operator4/1 -> Cout/1
  Cin/1 -> Logical Operator2/1, Logical Operator1/2
  Logical Operator2/1 -> Logical Operator4/1
  A/1 -> Logical Operator3/2, Logical Operator/1

== system Processor/Program Counter/Adder/Subsystem3 ==
  A : Inport
  B : Inport  Port=2
  Cin : Inport  Port=3
  Logical Operator : Logic  Operator=XOR  IconShape=distinctive  AllPortsSameDT=off  OutDataTypeStr=boolean
  Logical Operator1 : Logic  Operator=XOR  IconShape=distinctive  AllPortsSameDT=off  OutDataTypeStr=boolean
  Logical Operator2 : Logic  IconShape=distinctive  AllPortsSameDT=off  OutDataTypeStr=boolean
  Logical Operator3 : Logic  IconShape=distinctive  AllPortsSameDT=off  OutDataTypeStr=boolean
  Logical Operator4 : Logic  Operator=OR  IconShape=distinctive  AllPortsSameDT=off  OutDataTypeStr=boolean
  Sum : Outport
  Cout : Outport  Port=2
  wires:
  B/1 -> Logical Operator3/1, Logical Operator/2
  Logical Operator1/1 -> Sum/1
  Logical Operator3/1 -> Logical Operator4/2
  Logical Operator/1 -> Logical Operator2/2, Logical Operator1/1
  Logical Operator4/1 -> Cout/1
  Cin/1 -> Logical Operator2/1, Logical Operator1/2
  Logical Operator2/1 -> Logical Operator4/1
  A/1 -> Logical Operator3/2, Logical Operator/1

== stateflow chart Processor/Chart ==
  state Start
    PCenable=0;InstrRegEn=0;DecoderEnable=0;ALUenable=0;RegisterWriteEnable=0;
  state Fetch
    PCenable=1;InstrRegEn=1;DecoderEnable=0;ALUenable=0;RegisterWriteEnable=0;
  state timerresetate
    PCenable=0;InstrRegEn=0;DecoderEnable=0;ALUenable=0;RegisterWriteEnable=0;timerreset=1;
  state Decode
    PCenable=0;InstrRegEn=0;DecoderEnable=1;ALUenable=0;RegisterWriteEnable=0;
  state Execute
    PCenable=0;InstrRegEn=0;DecoderEnable=0;ALUenable=1;RegisterWriteEnable=0;
  state Writeback
    PCenable=0;InstrRegEn=0;DecoderEnable=0;ALUenable=0;RegisterWriteEnable=1;
  (default) -> Start
  Start -> Fetch
  timerresetate -> Fetch
  Fetch -> Decode : [delay>10]
  Writeback -> timerresetate : [delay>40]
  Decode -> Execute : [delay>20]
  Execute -> Writeback : [delay>30]
  data: delay input; PCenable output; DecoderEnable output; ALUenable output; RegisterWriteEnable output; InstrRegEn output; timerreset output
